simulink model "EV_simulation0x2DSwiftDesire"  (R2024b)
settings: Solver=VariableStepAuto  StartTime=0.0  StopTime=500  RelTol=1e-3
undefined symbols (not defined in the file): magnitude
settings Model: Creator=brain  LastModifiedBy=brain
settings DataIOCC: Refine=50

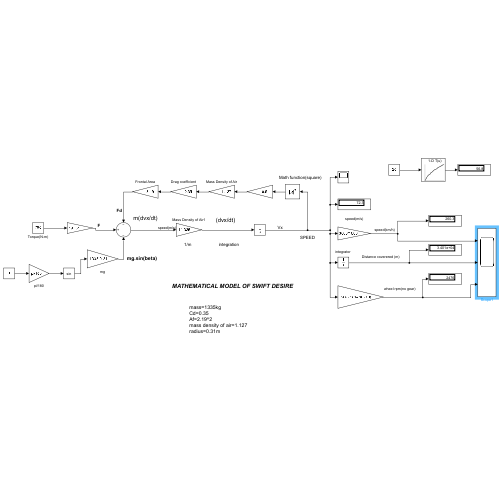
[thumbnail: Simulink's stored preview of the top-level diagram]
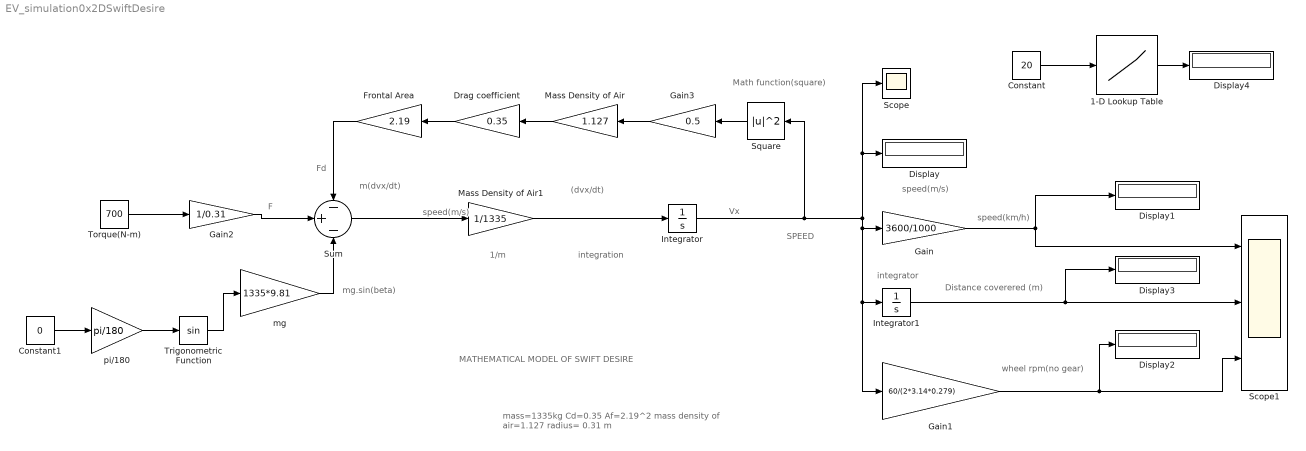
== system EV_simulation0x2DSwiftDesire ==
  note: Fd
  note: F
  note: speed(m/s)
  note: integration
  note: Vx
  note: SPEED
  note: 1/m
  note: Math function(square)
  note: m(dvx/dt)
  note: MATHEMATICAL MODEL OF SWIFT DESIRE
  note: mass=1335kg
      | Cd=0.35
      | Af=2.19^2
      | mass density of air=1.127
      | radius= 0.31 m
  note: mg.sin(beta)
  note: speed(km/h)
  note: Distance coverered (m)
  note: integrator
  note: wheel rpm(no gear)
  note: speed(m/s)
  note: (dvx/dt)
  1-D Lookup Table : Lookup_n-D  NumberOfTableDimensions=1  BreakpointsForDimension1=[5 10 15 20 25 30 35 40 45 50 55 60 65 70 75 80 85 90 95 100]  Table=[28.4 40.16 49.19 56.8 63.5 69.56 75.13 80.32 85.19 89.8 94.19 98.37 102.4 106.3 110 113.6 117.1 120.5 123.8 127]  InternalRulePriority=Speed  RndMeth=Simplest
  Constant : Constant  Value=20
  Constant1 : Constant  Value=0
  Display{,1..4} (5 alike) : Display
  Drag coefficient : Gain  Gain=0.35
  Frontal Area : Gain  Gain=2.19
  Gain : Gain  Gain=3600/1000
  Gain1 : Gain  Gain=60/(2*3.14*0.279)
  Gain2 : Gain  Gain=1/0.31
  Gain3 : Gain  Gain=0.5
  Integrator : Integrator
  Integrator1 : Integrator
  Mass Density of Air : Gain  Gain=1.127
  Mass Density of Air1 : Gain  Gain=1/1335
  Scope : Scope
  Scope1 : Scope  NumInputPorts=3
  Square : Math  Operator=magnitude^2
  Sum : Sum  Inputs=-+-
  Torque(N-m) : Constant  Value=700
  Trigonometric Function : Trigonometry
  mg : Gain  Gain=1335*9.81
  pi/180 : Gain  Gain=pi/180
  wires:
  Trigonometric Function/1 -> mg/1
  mg/1 -> Sum/3
  Frontal Area/1 -> Sum/1
  Square/1 -> Gain3/1
  Gain3/1 -> Mass Density of Air/1
  Mass Density of Air/1 -> Drag coefficient/1
  Drag coefficient/1 -> Frontal Area/1
  Sum/1 -> Mass Density of Air1/1
  Mass Density of Air1/1 -> Integrator/1
  Integrator/1 -> Scope/1, Display/1, Gain1/1, Integrator1/1, Gain/1, Square/1
  Gain1/1 -> Scope1/3, Display2/1
  Integrator1/1 -> Scope1/2, Display3/1
  Gain/1 -> Scope1/1, Display1/1
  Gain2/1 -> Sum/2
  Constant/1 -> 1-D Lookup Table/1
  1-D Lookup Table/1 -> Display4/1
  pi/180/1 -> Trigonometric Function/1
  Constant1/1 -> pi/180/1
  Torque(N-m)/1 -> Gain2/1
